simulink model "task2"  (R2024a)
settings: Solver=ode45  StartTime=0.0  StopTime=10  FixedStep=0.01  MaxStep=0.01  RelTol=1e-3
undefined symbols (not defined in the file): A, C, L, x0, x0_hat
settings Model: Creator=sizgr  LastModifiedBy=sizgr

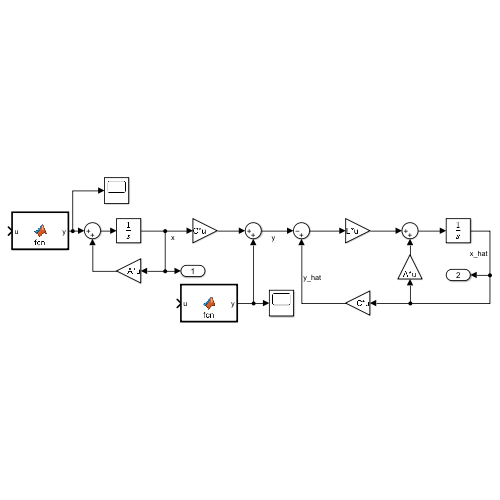
[thumbnail: Simulink's stored preview of the top-level diagram]
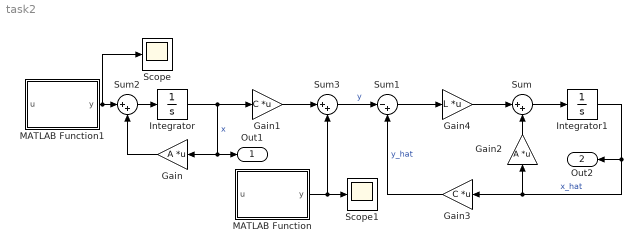
== system task2 ==
  Gain : Gain  Gain=A  Multiplication=Matrix(K*u)
  Gain1 : Gain  Gain=C  Multiplication=Matrix(K*u)
  Gain2 : Gain  Gain=A  Multiplication=Matrix(K*u)
  Gain3 : Gain  Gain=C  Multiplication=Matrix(K*u)
  Gain4 : Gain  Gain=L  Multiplication=Matrix(K*u)
  Integrator : Integrator  InitialCondition=x0
  Integrator1 : Integrator  InitialCondition=x0_hat
  MATLAB Function : MATLAB Function  TreatAsAtomicUnit=on
  MATLAB Function1 : MATLAB Function  TreatAsAtomicUnit=on
  Scope : Scope
  Scope1 : Scope
  Sum : Sum  Inputs=|++
  Sum1 : Sum  Inputs=|-+
  Sum2 : Sum  Inputs=|++
  Sum3 : Sum  Inputs=|++
  Out1 : Outport
  Out2 : Outport  Port=2
  wires:
  Integrator/1 -> Out1/1, Gain/1, Gain1/1  "x"
  Gain/1 -> Sum2/2
  Gain2/1 -> Sum/2
  Integrator1/1 -> Out2/1, Gain2/1, Gain3/1  "x_hat"
  Sum/1 -> Integrator1/1
  Gain3/1 -> Sum1/2  "y_hat"
  Sum1/1 -> Gain4/1
  Gain4/1 -> Sum/1
  Sum2/1 -> Integrator/1
  MATLAB Function1/1(y) -> Scope/1, Sum2/1
  Gain1/1 -> Sum3/1
  Sum3/1 -> Sum1/1  "y"
  MATLAB Function/1(y) -> Sum3/2, Scope1/1

== matlab function task2/MATLAB Function ==
  data: u input; y output
function y = fcn(u)

y = mvnrnd(zeros(1, 1), 1, 1);

== matlab function task2/MATLAB Function1 ==
  data: u input; y output
function y = fcn(u)

y = mvnrnd(zeros(1, 4), eye(4), 1)';
